simulink model "untitled"  (R2016b)
settings: Solver=FixedStepDiscrete  StartTime=0.0  StopTime=0.001  RelTol=1e-3
settings Model: Creator=mma137421  LastModifiedBy=mma137421
settings SolverCC: AutoInsertRateTranBlk=on
settings DataIOCC: LimitDataPoints=on  SaveOutput=off  SignalLogging=off  SaveTime=off
settings OptimizationCC: LifeSpan=inf
settings DebuggingCC: AlgebraicLoopMsg=error  SingleTaskRateTransMsg=error  AllowSymbolicDim=off  SFUnexpectedBacktrackingDiag=warning  SFNoUnconditionalDefaultTransitionDiag=warning  SFExecutionAtInitializationDiag=none
settings GRTTargetCC: TargetLangStandard=C89/C90 (ANSI)  GeneratePreprocessorConditionals=Disable all

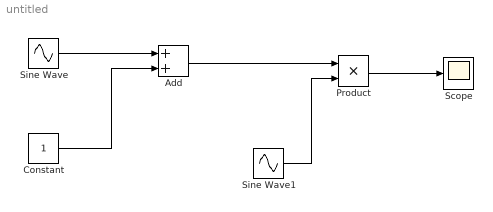
== system untitled ==
  Add : Sum
  Constant : Constant
  Product : Product
  Scope : Scope
  Sine Wave : Sin  Amplitude=2  Frequency=2*pi/0.0002  Phase=pi/2  SampleTime=0
  Sine Wave1 : Sin  Frequency=2*pi/0.00001  Phase=pi/2  SampleTime=0
  wires:
  Constant/1 -> Add/2
  Sine Wave/1 -> Add/1
  Add/1 -> Product/1
  Sine Wave1/1 -> Product/2
  Product/1 -> Scope/1
